simulink model "CH_humanoid_walker_rl_ARMS_REAL"  (R2021a)
settings: Solver=daessc  StartTime=0.0  StopTime=params.simulation.Tf  RelTol=1e-3  AbsTol=1e-3
model workspace (MATLAB code in the model file):
  | %% Humanoid Walker With Reinforcement Learning Intialization
  | % Copyright 2019 The MathWorks, Inc.
  | 
  | %% Joint rotation limits
  | %These limits are similar to human joint rotation limits.
  | 
  | % Legs joints
  | params.jointLimits.hipFrontalUpperLimit  =  30;  % (Deg)
  | params.jointLimits.hipFrontalLowerLimit  = -90;  % (Deg)
  | params.jointLimits.kneeUpperLimit        =  90;  % (Deg)
  | params.jointLimits.kneeLowerLimit        =  5;   % (Deg)
  | params.jointLimits.ankleUpperLimit       =  20;  % (Deg)
  | params.jointLimits.ankleLowerLimit       = -20;  % (Deg)
  | % Arm joints
  | params.jointLimits.shoulderFrontalUpperLimit        =  110; % (Deg)
  | params.jointLimits.shoulderFrontalLowerLimit        = -30;  % (Deg)
  | params.jointLimits.shoulderSagittalUpperLimit       =  90;  % (Deg)
  | params.jointLimits.shoulderSagittalLowerLimit       = -30;  % (Deg)
  | params.jointLimits.elbowLowerLimit                  = 5;    % (Deg)
  | params.jointLimits.elbowUpperLimit                  = 130;  % (Deg)
  | params.jointLimits.wristLowerLimit                  = -90;  % (Deg)
  | params.jointLimits.wristUpperLimit                  = 70;   % (Deg)
  | 
  | %% Motor Parameters: Left
  | % Current motor: https://uk.rs-online.com/web/p/dc-motors/7736804
  | %Stall Torque
  | params.motor.StallTorque.LeftHip                        = 100; % (Nm)
  | params.motor.StallTorque.LeftKnee                       = 100; % (Nm)
  | params.motor.StallTorque.LeftAnkle                      = 100; % (Nm)
  | 
  | params.motor.StallTorque.LeftShoulderFrontal            = 100; % (Nm)
  | params.motor.StallTorque.LeftShoulderSagital            = 100; % (Nm)
  | params.motor.StallTorque.LeftElbow                      = 100; % (Nm)
  | params.motor.StallTorque.LeftWrist                      = 100; % (Nm)
  | 
  | %Armature Inductance: UNKNOWN
  | params.motor.ArmatureInductance.LeftHip                 = 12e-6;
  | params.motor.ArmatureInductance.LeftKnee                = 12e-6;
  | params.motor.ArmatureInductance.LeftAnkle               = 12e-6;
  | 
  | params.motor.ArmatureInductance.LeftShoulderFrontal     = 12e-6;
  | params.motor.ArmatureInductance.LeftShoulderSagital     = 12e-6;
  | params.motor.ArmatureInductance.LeftElbow               = 12e-6;
  | params.motor.ArmatureInductance.LeftWrist               = 12e-6;
  | 
  | %No-Load Speed
  | params.motor.NoLoadSpeed.LeftHip                        = 22.5; % (RPM)
  | params.motor.NoLoadSpeed.LeftKnee                       = 22.5; % (RPM)
  | params.motor.NoLoadSpeed.LeftAnkle                      = 22.5; % (RPM)
  | 
  | params.motor.NoLoadSpeed.LeftShoulderFrontal            = 22.5; % (RPM)
  | params.motor.NoLoadSpeed.LeftShoulderSagital            = 22.5; % (RPM)
  | params.motor.NoLoadSpeed.LeftElbow                      = 22.5; % (RPM)
  | params.motor.NoLoadSpeed.LeftWrist                      = 22.5; % (RPM)
  | 
  | %Torque Constant
  | params.motor.RatedDCSupply.LeftHip                      = 12; % (V)
  | params.motor.RatedDCSupply.LeftKnee                     = 12; % (V)
  | params.motor.RatedDCSupply.LeftAnkle                    = 12; % (V)
  | 
  | params.motor.RatedDCSupply.LeftShoulderFrontal          = 12; % (V)
  | params.motor.RatedDCSupply.LeftShoulderSagital          = 12; % (V)
  | params.motor.RatedDCSupply.LeftElbow                    = 12; % (V)
  | params.motor.RatedDCSupply.LeftWrist                    = 12; % (V)
  | 
  | %% Motor Parameters: Right
  | %Stall Torque
  | params.motor.StallTorque.RightHip                        = 100; % (Nm)
  | params.motor.StallTorque.RightKnee                       = 100; % (Nm)
  | params.motor.StallTorque.RightAnkle                      = 100; % (Nm)
  | 
  | params.motor.StallTorque.RightShoulderFrontal            = 100; % (Nm)
  | params.motor.StallTorque.RightShoulderSagital            = 100; % (Nm)
  | params.motor.StallTorque.RightElbow                      = 100; % (Nm)
  | params.motor.StallTorque.RightWrist                      = 100; % (Nm)
  | 
  | %Armature Inductance
  | params.motor.ArmatureInductance.RightHip                 = 12e-6;
  | params.motor.ArmatureInductance.RightKnee                = 12e-6;
  | params.motor.ArmatureInductance.RightAnkle               = 12e-6;
  | 
  | params.motor.ArmatureInductance.RightShoulderFrontal     = 12e-6;
  | params.motor.ArmatureInductance.RightShoulderSagital     = 12e-6;
  | params.motor.ArmatureInductance.RightElbow               = 12e-6;
  | params.motor.ArmatureInductance.RightWrist               = 12e-6;
  | 
  | %No-Load Speed
  | params.motor.NoLoadSpeed.RightHip                        = 22.5; % (RPM)
  | params.motor.NoLoadSpeed.RightKnee                       = 22.5; % (RPM)
  | params.motor.NoLoadSpeed.RightAnkle                      = 22.5; % (RPM)
  | 
  | params.motor.NoLoadSpeed.RightShoulderFrontal            = 22.5; % (RPM)
  | params.motor.NoLoadSpeed.RightShoulderSagital            = 22.5; % (RPM)
  | params.motor.NoLoadSpeed.RightElbow                      = 22.5; % (RPM)
  | params.motor.NoLoadSpeed.RightWrist                      = 22.5; % (RPM)
  | 
  | %Torque Constant
  | params.motor.RatedDCSupply.RightHip                      = 12; % (V)
  | params.motor.RatedDCSupply.RightKnee                     = 12; % (V)
  | params.motor.RatedDCSupply.RightAnkle                    = 12; % (V)
  | 
  | params.motor.RatedDCSupply.RightShoulderFrontal          = 12; % (V)
  | params.motor.RatedDCSupply.RightShoulderSagital          = 12; % (V)
  | params.motor.RatedDCSupply.RightElbow                    = 12; % (V)
  | params.motor.RatedDCSupply.RightWrist                    = 12; % (V)
  | 
  | 
  | %% Material properties
  | 
  | params.materialProperties.lowerBodyDensity = 990;  % (kg/m^3)
  | params.materialProperties.upperBodyDensity = 1900; % (kg/m^3)
  | 
  | %% World damping
  | % We add damping to the vertical (z) and rotational (Rx, Ry, Rz) components
  | % of the bushing joint. This dissipates energy from the system and facilates
  | % quicker learning. Increasing this improves stability and learning, but is
  | % less realistic.
  | 
  | params.simulation.worldDamping = 6; % (Ns/m)
  | 
  | %% Simulation parameters
  | 
  | params.simulation.initialHeight=1.54; % (m) Intial height of robot
  | params.simulation.Ts = 0.025;         % (s) Control and sensing discretization time
  | params.simulation.Tf = 600;      % (s) Max simulation time
  | 
  | %% Spatial contact force block parameters.
  | % The value of these parameters affects simulation and learning speed.
  | % Higher damping generally improves learning but slows down simulation.
  | % High static and dynamic friction values tend to improve learning.
  | 
  | params.contact.stiffness        = 1e5;  % (N/m)
  | params.contact.damping          = 1e5;  % (Ns/m)
  | params.contact.transitionWidth  = 1e-3; % (m)
  | params.contact.staticFriction   = 1;    % ()
  | params.contact.dynamicFriction  = 0.9;  % ()
  | params.contact.criticalVelocity = 1e-3; % (m/s)
  | params.contact.contactRadius = 0.01;    % (m)
  | 
  | %% Controller parameters
  | 
  | params.controller.hipFrontalStiffness  = 80; % (N*m/rad)
  | params.controller.hipFrontalDamping    = 1;  % (N*m*s/rad)
  | params.controller.kneeStiffness        = 80; % (N*m*/rad)
  | params.controller.kneeDamping          = 1;  % (N*m*s/rad)
  | params.controller.ankleStiffness       = 80; % (N*m/rad)
  | params.controller.ankleDamping         = 1;  % (N*m*s/rad)
  | 
  | 
  | %% Stopping criteria
  | % Define the conditions under which the simulation is terminated early.
  | % One or more of three conditions need to be satisfied for termination.
  | % If the humanoid torso drops vertically, travels laterally or rotates in
  | % any axis more than a set of predefined values, or if the humanoid stops
  | % moving.
  | 
  | params.stoppingCriteria.forward          = 4;   % (m)
  | params.stoppingCriteria.lateral          = 4;   % (m)
  | params.stoppingCriteria.angle            = 45;  % (deg)
  | params.stoppingCriteria.timeoutTime      = 2;   % (s)
  | params.stoppingCriteria.timeoutDistance  = 0.5;   % (m)
  | 
  | %% Reward scaling parameters
  | 
  | params.reward.forwardPenaltyWeight   = 15;    % Forward velocity scale, w_1
  | params.reward.timestepRewardWeight  = 1;    % Not falling scale, w_2
  | params.reward.powerPenaltyWeight    = 5e-4; % Power scale, w_3
  | params.reward.verticalRewardWeight = 50;   % Vertical displacement scale, w_4
  | params.reward.lateralPenaltyWeight  = 15;  % Lateral displacement scale, w_5
  | 
  | %% Display parameters
  | 
  | params.display.tileColour    = [0.956, 0.941, 0.941];
  | params.display.floorColour   = [0.756, 0.741, 0.741];
  | params.display.tileThickness = 0.005;
  | params.display.planeWidth        = 5;   % (m)
  | params.display.planeLength       = 5;  % (m)
  | params.display.planeHeight       = 1;   % (m)
  | params.display.Gravity           = [0, 0, -9.80665];   % (m/s^2)
undefined symbols (not defined in the file or in its folder): rl
libraries: CH_Library x4, sm_lib x3, nesl_utility x1, rllib x1
settings Model: Creator=The MathWorks, Inc.  LastModifiedBy=coa19cdd
settings SolverCC: AlgebraicLoopSolver=TrustRegion
settings DebuggingCC: SolverPrmCheckMsg=warning  ParameterPrecisionLossMsg=none  ParameterTunabilityLossMsg=none  StateNameClashWarn=warning  SFMachineParentedDataDiag=warning
settings ExplorerConfigSet: InternalSimMechanicsExplorerSettings="<ExplorerConfiguration><canonicalview>default</canonicalview><AnimationSetting><BasePlaybackSpeed>1.0</BasePlaybackSpeed><PlaybackSpeedFactor>1.0</PlaybackSpeedFactor></AnimationSetting><TilePanel><TileInfo><Tiles Columns=\"1\" Count=\"1\" Rows=\"1\"><Column Weight=\"1\"/><Row Weight=\"1\"/><Tile Height=\"1\" Width=\"1\" X=\"0\" Y=\"0\"/></Tiles></TileInfo><SceneInfo><SceneViewer><BGColor><R>0.800000011920928955</R><G>1</G><B>1</B></BGColor><Camera><DoPerspective>on</DoPerspective><Position><X>-3.97064206882887039</X><Y>-26.3666352607981089</Y><Z>2.92141226580509095</Z></Position><Center><X>-0.00178258174571515032</X><Y>-23.3217627759063362</Y><Z>1.933026752688358</Z></Center><Up><X>0</X><Y>0</Y><Z>1</Z></Up><ViewLimDist>1</ViewLimDist><YLim>0.466307658154998583</YLim><XLim>0.727439946721797792</XLim></Camera></SceneViewer></SceneInfo></TilePanel><MechEditorPanel><Cameras><Camera><Id>Camera1</Id><Value><Name>Camera1</Name><NativeCamera><PositionTrackingFeature>Humanoid_Walker.Humanoid_Robot_6_Joint.Camera_Frame.R</PositionTrackingFeature><CenterTrackingFeature>Humanoid_Walker.Humanoid_Robot_6_Joint.Aim_Frame.R</CenterTrackingFeature><UpVectorTrackingFeature>Humanoid_Walker.Humanoid_Robot_6_Joint.World.W</UpVectorTrackingFeature><CenterTrackingOrigin>on</CenterTrackingOrigin><UpVectorTrackingDirection>+Z</UpVectorTrackingDirection></NativeCamera></Value></Camera><Camera><Id>Camera2</Id><Value><Name>IT FOLLOWS ME HOME</Name><NativeCamera><PositionTrackingFeature>Learning_Environment.Physical_Model.Humanoid_Robot.Torso_and_Head.Camera.Spherical_Solid.R</PositionTrackingFeature><CenterTrackingFeature>Learning_Environment.Physical_Model.Humanoid_Robot.Torso_and_Head.Camera.Camera_Rotation.F</CenterTrackingFeature><UpVectorTrackingFeature>Learning_Environment.Physical_Model.World_Frame.W</UpVectorTrackingFeature><CenterTrackingOrigin>on</CenterTrackingOrigin><UpVectorTrackingDirection>+Z</UpVectorTrackingDirection></NativeCamera></Value></Camera></Cameras><GfxPanelCameraMap><MapElement CameraMLId=\"Camera2\" GfxPanelIndex=\"0\"/></GfxPanelCameraMap><VideoCreator><PlaybackSpeedRatio>1.0</PlaybackSpeedRatio><FrameRate>30</FrameRate><VideoFormat>Motion JPEG AVI</VideoFormat><FrameSize>auto</FrameSize></VideoCreator></MechEditorPanel></ExplorerConfiguration>"

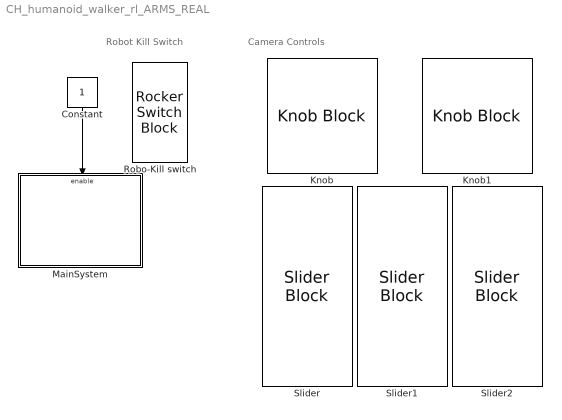
== system CH_humanoid_walker_rl_ARMS_REAL ==
  note: Camera Controls
  note: Robot Kill Switch
  Constant : Constant
  Knob : KnobBlock  ScaleMax=360  TickInterval=45
  Knob1 : KnobBlock  ScaleMax=360  TickInterval=45
  MainSystem : Subsystem
  Robo-Kill switch : RockerSwitchBlock  LabelPosition=Hide
      settings: Values={{'Alive', 'Dead'}, [1 -1]}
  Slider : SliderBlock  ScaleMax=5  TickInterval=1
  Slider1 : SliderBlock  ScaleMax=5  TickInterval=1
  Slider2 : SliderBlock  ScaleMax=5  TickInterval=1
  wires:
  Constant/1 -> MainSystem/Enable

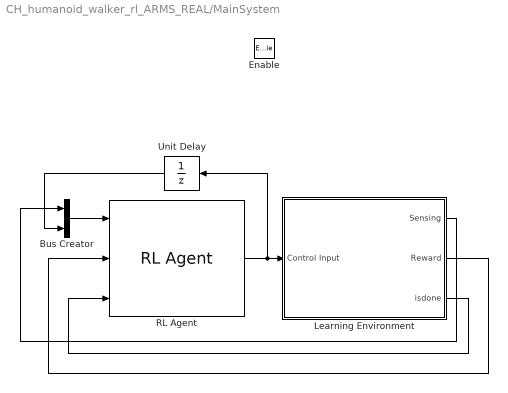
== system CH_humanoid_walker_rl_ARMS_REAL/MainSystem ==
  Enable : EnablePort  StatesWhenEnabling=reset  PropagateVarSize=During execution
  Bus Creator : BusCreator  Inputs=2
  Learning Environment : Subsystem
  RL Agent : rllib/RL Agent  Agent=rl.util.PolicyInstance.get()  ExternalActionAsInput=off  ProvideCumRwd=off  TreatAsDirectFeedthrough=on
  Unit Delay : UnitDelay  SampleTime=params.simulation.Ts  HasFrameUpgradeWarning=on
  wires:
  Learning Environment/1(Sensing) -> Bus Creator/1
  RL Agent/1 -> Unit Delay/1, Learning Environment/1(Control Input)
  Learning Environment/3(isdone) -> RL Agent/3
  Bus Creator/1 -> RL Agent/1
  Unit Delay/1 -> Bus Creator/2
  Learning Environment/2("Reward ") -> RL Agent/2

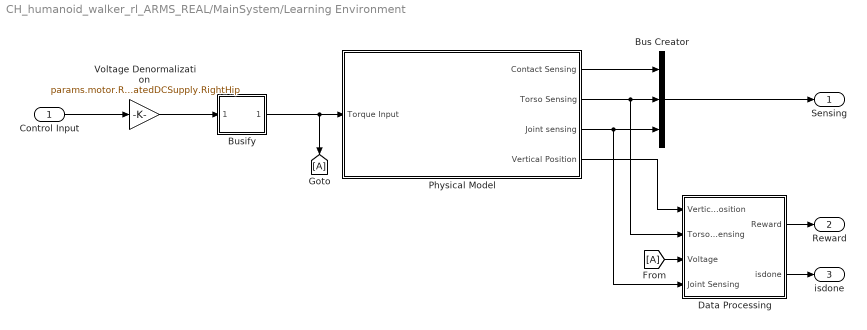
== system CH_humanoid_walker_rl_ARMS_REAL/MainSystem/Learning Environment ==
  Control Input : Inport
  Bus Creator : BusCreator  Inputs=3
  Busify : Subsystem
  Data Processing : Subsystem
  Physical Model : Subsystem
      mask Display: image('imagebackground.PNG'); % Use "Edit Image" on toolstrip to change.
  Voltage Denormalization : Gain  Gain=params.motor.RatedDCSupply.RightHip
  Sensing : Outport
  "Reward " : Outport  Port=2
  isdone : Outport  Port=3
  wires:
  Physical Model/1(Contact Sensing) -> Bus Creator/1
  Bus Creator/1 -> Sensing/1
  Physical Model/2(Torso Sensing) -> Data Processing/2(Torso Sensing), Bus Creator/2
  Physical Model/3(Joint sensing) -> Data Processing/4(Joint Sensing), Bus Creator/3
  [A] -> Data Processing/3(Voltage)
  Data Processing/1(Reward) -> "Reward "/1
  Data Processing/2(isdone) -> isdone/1
  Physical Model/4(Vertical Position) -> Data Processing/1(Vertical Position)
  Busify/1(Out1) -> [A], Physical Model/1(Torque Input)
  Control Input/1 -> Voltage Denormalization/1
  Voltage Denormalization/1 -> Busify/1(Control Input)

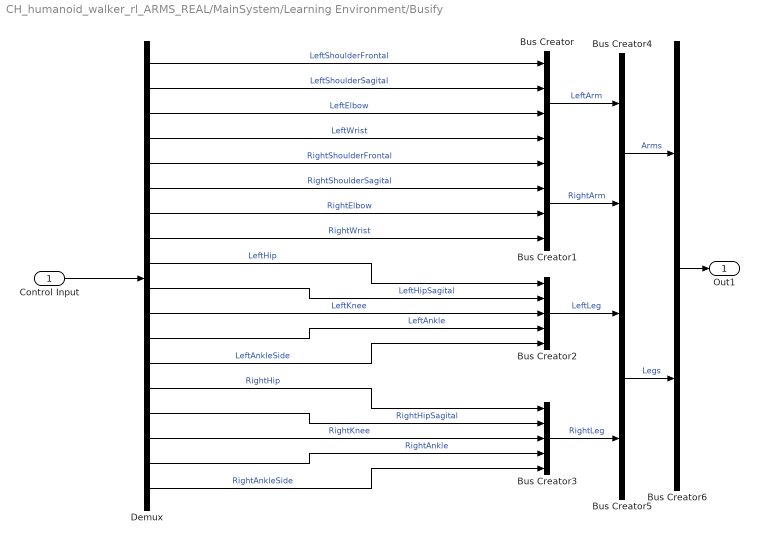
== system CH_humanoid_walker_rl_ARMS_REAL/MainSystem/Learning Environment/Busify ==
  Control Input : Inport
  Bus Creator : BusCreator  Inputs=4
  Bus Creator1 : BusCreator  Inputs=4
  Bus Creator2 : BusCreator  Inputs=5
  Bus Creator3 : BusCreator  Inputs=5
  Bus Creator4 : BusCreator  Inputs=2
  Bus Creator5 : BusCreator  Inputs=2
  Bus Creator6 : BusCreator  Inputs=2
  Demux : Demux  Outputs=18
  Out1 : Outport
  wires:
  Control Input/1 -> Demux/1
  Demux/1 -> Bus Creator/1  "LeftShoulderFrontal"
  Demux/2 -> Bus Creator/2  "LeftShoulderSagital"
  Demux/3 -> Bus Creator/3  "LeftElbow"
  Demux/4 -> Bus Creator/4  "LeftWrist"
  Demux/5 -> Bus Creator1/1  "RightShoulderFrontal"
  Demux/6 -> Bus Creator1/2  "RightShoulderSagital"
  Demux/7 -> Bus Creator1/3  "RightElbow"
  Demux/8 -> Bus Creator1/4  "RightWrist"
  Demux/9 -> Bus Creator2/1  "LeftHip"
  Demux/11 -> Bus Creator2/3  "LeftKnee"
  Demux/12 -> Bus Creator2/4  "LeftAnkle"
  Demux/14 -> Bus Creator3/1  "RightHip"
  Demux/16 -> Bus Creator3/3  "RightKnee"
  Demux/17 -> Bus Creator3/4  "RightAnkle"
  Bus Creator/1 -> Bus Creator4/1  "LeftArm"
  Bus Creator1/1 -> Bus Creator4/2  "RightArm"
  Bus Creator2/1 -> Bus Creator5/1  "LeftLeg"
  Bus Creator3/1 -> Bus Creator5/2  "RightLeg"
  Bus Creator4/1 -> Bus Creator6/1  "Arms"
  Bus Creator5/1 -> Bus Creator6/2  "Legs"
  Bus Creator6/1 -> Out1/1
  Demux/10 -> Bus Creator2/2  "LeftHipSagital"
  Demux/13 -> Bus Creator2/5  "LeftAnkleSide"
  Demux/15 -> Bus Creator3/2  "RightHipSagital"
  Demux/18 -> Bus Creator3/5  "RightAnkleSide"

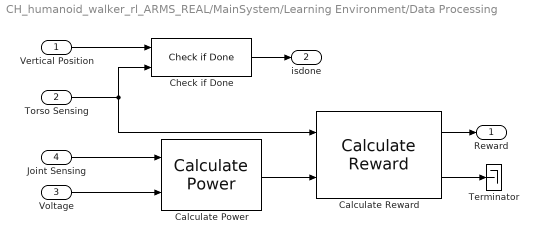
== system CH_humanoid_walker_rl_ARMS_REAL/MainSystem/Learning Environment/Data Processing ==
  Vertical Position : Inport
  Torso Sensing : Inport  Port=2
  Voltage : Inport  Port=3
  Joint Sensing : Inport  Port=4
  Calculate Power : CH_Library/Calculate Power  SystemSampleTime=-1  VariantActivationTime=update diagram  Latency=0  AutoFrameSizeCalculation=off
  Calculate Reward : CH_Library/Calculate Reward  forwardPenalty=params.reward.forwardPenaltyWeight  timestepReward=params.reward.timestepRewardWeight  powerPenalty=params.reward.powerPenaltyWeight  verticalReward=params.reward.verticalRewardWeight  lateralPenalty=params.reward.lateralPenaltyWeight
  Check if Done : CH_Library/Check if Done  forwardStop=params.stoppingCriteria.forward  lateralStop=params.stoppingCriteria.lateral  angularStop=params.stoppingCriteria.angle  timeoutTime=params.stoppingCriteria.timeoutTime  timeoutDistance=params.stoppingCriteria.timeoutDistance
  Terminator : Terminator
  Reward : Outport
  isdone : Outport  Port=2
  wires:
  Torso Sensing/1 -> Check if Done/2, Calculate Reward/1
  Check if Done/1 -> isdone/1
  Calculate Power/1 -> Calculate Reward/2
  Joint Sensing/1 -> Calculate Power/1
  Voltage/1 -> Calculate Power/2
  Calculate Reward/1 -> Reward/1
  Vertical Position/1 -> Check if Done/1
  Calculate Reward/2 -> Terminator/1

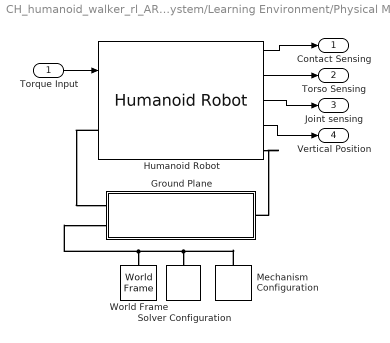
== system CH_humanoid_walker_rl_ARMS_REAL/MainSystem/Learning Environment/Physical Model ==
  Torque Input : Inport
  Ground Plane : Subsystem
  Humanoid Robot : CH_Library/Humanoid Robot  contactRadius=params.contact.contactRadius  contactStiffness=params.contact.stiffness  contactDamping=params.contact.damping  contactTWidth=params.contact.transitionWidth  contactStaticFriction=params.contact.staticFriction  contactDynamicFriction=params.contact.dynamicFriction  contactCriticalVelocity=params.contact.criticalVelocity  footDensity=params.materialProperties.lowerBodyDensity  lowerLegDensity=params.materialProperties.lowerBodyDensity  upperLegDensity=params.materialProperties.lowerBodyDensity  hipDensity=params.materialProperties.lowerBodyDensity  trunkDensity=params.materialProperties.upperBodyDensity  shoulderDensity=params.materialProperties.upperBodyDensity  upperArmDensity=params.materialProperties.upperBodyDensity  lowerArmDensity=params.materialProperties.upperBodyDensity  handDensity=params.materialProperties.upperBodyDensity  headDensity=params.materialProperties.upperBodyDensity  hipUpperLimit=params.jointLimits.hipFrontalUpperLimit  hipLowerLimit=params.jointLimits.hipFrontalLowerLimit  kneeUpperLimit=params.jointLimits.kneeUpperLimit  kneeLowerLimit=params.jointLimits.kneeLowerLimit  ankleUpperLimit=params.jointLimits.ankleUpperLimit  ankleLowerLimit=params.jointLimits.ankleLowerLimit  shoulderFrontalUpperLimit=params.jointLimits.shoulderFrontalUpperLimit  shoulderFrontalLowerLimit=params.jointLimits.shoulderFrontalLowerLimit  shoulderSagittalUpperLimit=params.jointLimits.shoulderSagittalUpperLimit  shoulderSagittalLowerLimit=params.jointLimits.shoulderSagittalLowerLimit  elbowUpperLimit=params.jointLimits.ankleUpperLimit  elbowLowerLimit=params.jointLimits.shoulderSagittalLowerLimit  wristUpperLimit=params.jointLimits.ankleUpperLimit  wristLowerLimit=params.jointLimits.shoulderSagittalLowerLimit
  Mechanism Configuration : sm_lib/Utilities/Mechanism Configuration  UniformGravity=Constant  GravityVector=[0, 0, -9.80665]  GravityVectorUnits=m/s^2  GravityUnits=m/s^2  LinearizationDelta=0.001  JointModeTransitionNonlinearIterations=2
  Solver Configuration : nesl_utility/Solver Configuration  PhysicalDomain=network_engine_domain  SubClassName=solver  LeftPortType=input  RightPortType=generic  Tones=[]  Harmonics=[]  SimulateNoise=off  Profile=off  UseLocalSampling=off  EnableSwitchedLinearOptims=on  FrequencyDomain=off  UseCCode=off  RelTol=0.001  AbsTol=1e-06  MinStep=1e-09  ToWorkspace=off  RevertToSquareIcSolve=off  NumHomotopyIterations=100  PhasorMode=off  PhasorModeNumHarmonics=1  DoDC=off  ResidualTolerance=1e-09  UseLocalSolver=off  LocalSolverChoice=NE_BACKWARD_EULER_ADVANCER  LocalSolverSampleTime=0.001  DoFixedCost=off  MaxNonlinIter=3  MaxModeIter=2  ComputeImpulses=off  ImpulseIterations=2  LinearAlgebra=Full  EquationFormulation=NE_TIME_EF  DelaysMemoryBudget=1024  AutomaticFiltering=on  FilteringTimeConstant=0.001  PartitionStorageMethod=AS_NEEDED  PartitionMemoryBudget=1024  PartitionMethod=ROBUST
      settings: SourceProductBaseCode=PW,SS
  World Frame : sm_lib/Frames and Transforms/World Frame
  Contact Sensing : Outport
  Torso Sensing : Outport  Port=2
  Joint sensing : Outport  Port=3
  Vertical Position : Outport  Port=4
  wires:
  Humanoid Robot/2 -> Torso Sensing/1
  Humanoid Robot/1 -> Contact Sensing/1
  Torque Input/1 -> Humanoid Robot/1
  Humanoid Robot/3 -> Joint sensing/1
  Humanoid Robot/4 -> Vertical Position/1
  connections:
  Humanoid Robot/RConn1 -- Ground Plane/RConn1
  Mechanism Configuration/RConn1 -- World Frame/RConn1 -- Ground Plane/LConn2 -- Solver Configuration/RConn1
  Humanoid Robot/LConn1 -- Ground Plane/LConn1

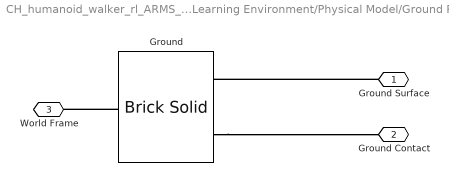
== system CH_humanoid_walker_rl_ARMS_REAL/MainSystem/Learning Environment/Physical Model/Ground Plane ==
  Ground : sm_lib/Body Elements/Brick Solid  GraphicAmbientColor=[0.15 0.15 0.15 1.0]  BasedOnType=Density  BrickDimensions=[params.display.planeWidth params.display.planeLength params.display.planeHeight]  BrickDimensionUnits=m  CenterOfMass=[0 0 0]  CenterOfMassUnits=m  GraphicDiffuseColor=params.display.floorColour  Density=1000  DensityUnits=kg/m^3  DoExposeReferenceFrame=on  GraphicEmissiveColor=[1.0 1.0 1.0 1.0]  ExportEntireGeometry=on  SerializedFrames=<Frames><Frame><Id>Frame1</Id><Value><Name>GS</Name><Origin><Source>GeometricFeature</Source><FeatureName>+z surface</FeatureName></Origin><PrimaryAxis><DefinedDirection>+Z</DefinedDirection><Source>ReferenceFrame</Source><SourceDirection>+Z</SourceDirection><FeatureName></FeatureName></PrimaryAxis><SecondaryAxis><DefinedDirection>+X</DefinedDirection><Source>ReferenceFrame</Source><SourceDirection>+X</SourceDirection><FeatureName></FeatureName></SecondaryAxis></Value></Frame></Frames>  MarkerShape=Sphere  MarkerSize=10  GraphicType=FromGeometry  InertiaType=CalculateFromGeometry  Mass=1  MassUnits=kg  MomentsOfInertia=[1 1 1]  MomentsOfInertiaUnits=kg*m^2  GraphicOpacity=0.3  ProductsOfInertia=[0 0 0]  ProductsOfInertiaUnits=kg*m^2  GraphicShininess=128  GraphicSpecularColor=[0.5 0.5 0.5 1.0]  GraphicVisPropType=SimpleVisualProperties
  Ground Surface : PMIOPort  Side=Left
  Ground Contact : PMIOPort  Port=2  Side=Right
  World Frame : PMIOPort  Port=3  Side=Left
  connections:
  Ground Surface/RConn1 -- Ground/LConn1
  Ground/LConn2 -- Ground Contact/RConn1
  Ground/RConn1 -- World Frame/RConn1
